simulink model "lab6_1"  (R2018a)
settings: Solver=ode45  StartTime=0.0  StopTime=100  MaxStep=0.001  RelTol=1e-3
settings Model: Creator=Koala  LastModifiedBy=Koala

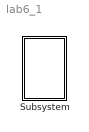
== system lab6_1 ==
  Subsystem : Subsystem  mask{Qwe=40, S1=1, S2=0.5, Swy1=1, Swy2=0.5, fi1=0.4, fi2=1}

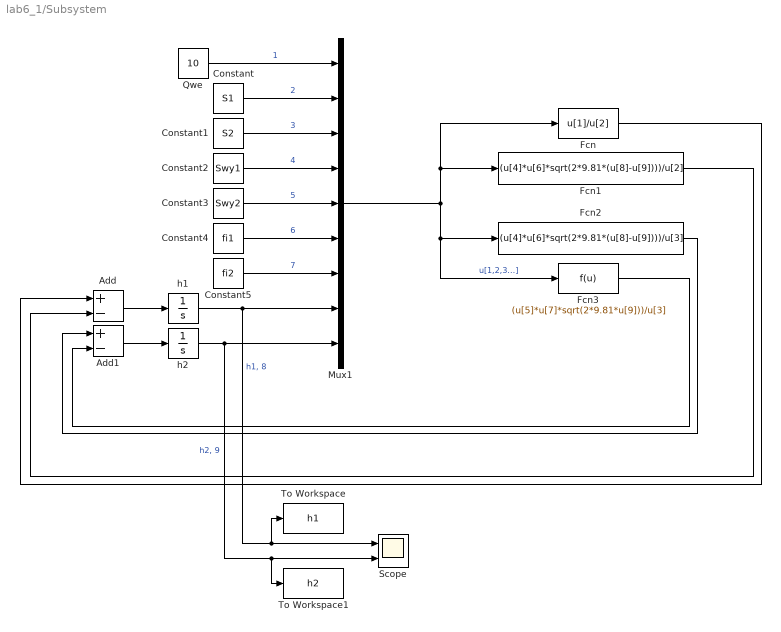
== system lab6_1/Subsystem ==
  Add : Sum  Inputs=+-
  Add1 : Sum  Inputs=+-
  Constant : Constant  Value=S1
  Constant1 : Constant  Value=S2
  Constant2 : Constant  Value=Swy1
  Constant3 : Constant  Value=Swy2
  Constant4 : Constant  Value=fi1
  Constant5 : Constant  Value=fi2
  Fcn : Fcn  Expr=u[1]/u[2]
  Fcn1 : Fcn  Expr=(u[4]*u[6]*sqrt(2*9.81*(u[8]-u[9])))/u[2]
  Fcn2 : Fcn  Expr=(u[4]*u[6]*sqrt(2*9.81*(u[8]-u[9])))/u[3]
  Fcn3 : Fcn  Expr=(u[5]*u[7]*sqrt(2*9.81*u[9]))/u[3]
  Mux1 : Mux  Inputs=9
  Qwe : Constant  Value=10
  Scope : Scope  NumInputPorts=2
  To Workspace : ToWorkspace  VariableName=h1  SampleTime=-1
  To Workspace1 : ToWorkspace  VariableName=h2  SampleTime=-1
  h1 : Integrator
  h2 : Integrator
  wires:
  Constant5/1 -> Mux1/7  "7"
  Constant4/1 -> Mux1/6  "6"
  Constant3/1 -> Mux1/5  "5"
  Constant2/1 -> Mux1/4  "4"
  Constant1/1 -> Mux1/3  "3"
  Constant/1 -> Mux1/2  "2"
  h1/1 -> To Workspace/1, Scope/1, Mux1/8  "h1, 8"
  h2/1 -> To Workspace1/1, Scope/2, Mux1/9  "h2, 9"
  Mux1/1 -> Fcn1/1, Fcn/1, Fcn3/1, Fcn2/1  "u[1,2,3...]"
  Qwe/1 -> Mux1/1  "1"
  Fcn/1 -> Add/1
  Fcn1/1 -> Add/2
  Add/1 -> h1/1
  Fcn2/1 -> Add1/1
  Fcn3/1 -> Add1/2
  Add1/1 -> h2/1
